simulink model "basic_simulink"  (R2020a)
settings: Solver=VariableStepAuto  StartTime=0.0  StopTime=10.0  RelTol=1e-3
settings Model: Creator=Pｈｉｌ  LastModifiedBy=Pｈｉｌ

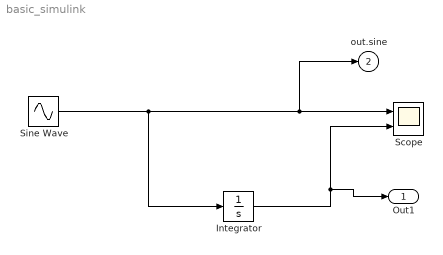
== system basic_simulink ==
  Integrator : Integrator
  Scope : Scope  NumInputPorts=2
  Sine Wave : Sin  SampleTime=0
  Out1 : Outport  SignalName=out.ints
  out.sine : Outport  Port=2  VectorParamsAs1DForOutWhenUnconnected=off
  wires:
  Sine Wave/1 -> Integrator/1, out.sine/1, Scope/1
  Integrator/1 -> Out1/1, Scope/2
